simulink model "ADCS_Outline"  (R2019a)
settings: Solver=VariableStepAuto  StartTime=0.0  StopTime=duration  MaxStep=step
InitFcn:
  | SC_ODIN_INITIALIZATION
values from neighbouring files (symbols this model uses):
  A = [ v(1) v(4) v(5) v(7);        v(4) v(2) v(6) v(8);        v(5) v(6) v(3) v(9);        v(7) v(8) v(9) v(10) ]    [MagnetometerCalibration.m]    (also in SC_ODIN_INITIALIZATION.m = 0.06; test.m = asin(sin(N)/sin(n)*sin(a)))
  Amag = [0.910186583854  -0.00959593267728  0.00343590491018; -0.00959593267728  1.05471221352  0.0559849466324; 0.00343590491018  0.0559849466324  1.05528532305]    [MagnetometerBias.mat]    (also in MagnetometerCalibration.m = evecs/scale*evecs')
  argentina = [1612.36;-4182.16;-4522.83]    [SC_ODIN_INITIALIZATION.m]
  As = 0.2*0.3    (= 0.06)    [SC_ODIN_INITIALIZATION.m]
  b_mag = block.InputPort(3).Data    [MagnetometerCalibration.m]    (also in SC_ODIN_INITIALIZATION.m = [10;-15.5;-12.2]*1e-6)
  bmag = [1.00003671399e-05 -1.55007781395e-05 -1.22009762149e-05]    [MagnetometerBias.mat]    (also in MagnetometerCalibration.m = centerE)
  breakpoints = data(:,1)    [SC_ODIN_INITIALIZATION.m]
  c = 2.99792458e8    (= 299792458)    [SC_ODIN_INITIALIZATION.m]
  C_I = [0.045 0.0009 -0.00007;        0.0009 0.045 -0.00003;        -0.00007 -0.00003 0.009]    [SC_ODIN_INITIALIZATION.m]
  Cd = 2.0    (= 2)    [SC_ODIN_INITIALIZATION.m]
  controller_sample_rate = 0.5    [SC_ODIN_INITIALIZATION.m]
  D = [ 2 * x,            2 * y,            2 * z,            1 + 0 * x ]    [MagnetometerCalibration.m]    (also in SC_ODIN_INITIALIZATION.m = 0.01*[1;1;1])
  datapx = data(:,2)    [SC_ODIN_INITIALIZATION.m]
  datapy = data(:,3)    [SC_ODIN_INITIALIZATION.m]
  datapz = data(:,4)    [SC_ODIN_INITIALIZATION.m]
  datavx = data(:,5)    [SC_ODIN_INITIALIZATION.m]
  datavy = data(:,6)    [SC_ODIN_INITIALIZATION.m]
  datavz = data(:,7)    [SC_ODIN_INITIALIZATION.m]
  DCM_BT0 = eye(3)    [SC_ODIN_INITIALIZATION.m]
  G = 6.67408e-11    [SC_ODIN_INITIALIZATION.m]
  ground = [1266.06;-4295.81;4526.14]    [SC_ODIN_INITIALIZATION.m]
  I = [Ixx -Ixy -Ixz;      -Ixy Iyy -Iyz;      -Ixz -Iyz Izz]    [SC_ODIN_INITIALIZATION.m]
  invA_mag = block.InputPort(2).Data    [MagnetometerCalibration.m]    (also in SC_ODIN_INITIALIZATION.m = inv(Ellrot/scale*Ellrot'))
  JD_0 = start_day+start_fraction    [SC_ODIN_INITIALIZATION.m]
  Ks = 1367    [SC_ODIN_INITIALIZATION.m]
  L = [0.0000812 -0.0022136 -0.0225868]    [SC_ODIN_INITIALIZATION.m]
  Ls = 0.01*[-3; 3; 5]    [SC_ODIN_INITIALIZATION.m]
  M = 5.9722e24    (= 5.9722e+24)    [SC_ODIN_INITIALIZATION.m]    (also in visualisation.m = uicontrol('Style','text','String',{''},'Position',[710 100+2)
  magnetorquer_tau = 0.02    [SC_ODIN_INITIALIZATION.m]
  magnetorquer_x_saturation = 0.24    [SC_ODIN_INITIALIZATION.m]
  magnetorquer_y_saturation = 0.24    [SC_ODIN_INITIALIZATION.m]
  magnetorquer_z_saturation = 0.13    [SC_ODIN_INITIALIZATION.m]
  namibia = [5659.26;1238.85;-2659.2]    [SC_ODIN_INITIALIZATION.m]
  q = 0.6    [SC_ODIN_INITIALIZATION.m]
  radii = radii .* sgns    [MagnetometerCalibration.m]    (also in SC_ODIN_INITIALIZATION.m = [1;0.9;1.1])
  W0 = [1;0;1-1/240].*pi()/180    [SC_ODIN_INITIALIZATION.m]
  wheel_saturation = 0.23e-3    (= 0.00023)    [SC_ODIN_INITIALIZATION.m]
  wheel_tau = 2    [SC_ODIN_INITIALIZATION.m]
undefined symbols (not defined in the file or in its folder): DiscIntNeverNeededParam, nut80, sun_sensors
libraries: dspmathops x94, vrlib x70, dspsrcs4 x21, realtime_pacer_lib x1, dspsolvers x1, dspinverses x1
(part 4 of 6)

== matlab function ADCS_Outline/SGP4/SGP4 ==
  data: TT input; pos output size=3; vel output size=3
function [pos , vel] = SGP4(TT)
ge = 398600.8; % Earth gravitational constant
TWOPI = 2*pi;
MINUTES_PER_DAY = 1440.0;
MINUTES_PER_DAY_SQUARED = (MINUTES_PER_DAY * MINUTES_PER_DAY);
MINUTES_PER_DAY_CUBED = (MINUTES_PER_DAY * MINUTES_PER_DAY_SQUARED);

% TLE file
% ISS (ZARYA)             
% 1 25544U 98067A   19233.64704772  .00000489  00000-0  16413-4 0  9995
% 2 25544  51.6448  36.5251 0007392 309.8359 134.3211 15.50389354185417
tle1 = '1 25544U 98067A   19233.64704772  .00000489  00000-0  16413-4 0  9995';
tle2 = '2 25544  51.6448  36.5251 0007392 309.8359 134.3211 15.50389354185417';


% Open the TLE file and read TLE elements


% 19-32	04236.56031392	Element Set Epoch (UTC)
% 3-7	25544	Satellite Catalog Number
% 9-16	51.6335	Orbit Inclination (degrees)
% 18-25	344.7760	Right Ascension of Ascending Node (degrees)
% 27-33	0007976	Eccentricity (decimal point assumed)
% 35-42	126.2523	Argument of Perigee (degrees)
% 44-51	325.9359	Mean Anomaly (degrees)
% 53-63	15.70406856	Mean Motion (revolutions/day)
% 64-68	32890	Revolution Number at Epoch

    % read first line
    tline = tle1;

    Cnum = tline(3:7);      			        % Catalog Number (NORAD)
    SC   = tline(8);					        % Security Classification
    ID   = tline(10:17);			            % Identification Number
    epoch = str2double(tline(19:32));              % Epoch
    TD1   = str2double(tline(34:43));              % first time derivative
    TD2   = str2double(tline(45:50));              % 2nd Time Derivative
    ExTD2 = tline(51:52);                       % Exponent of 2nd Time Derivative
    BStar = str2double(tline(54:59));              % Bstar/drag Term
    ExBStar = str2double(tline(60:61));            % Exponent of Bstar/drag Term
    BStar = BStar*1e-5*10^ExBStar;
    Etype = tline(63);                          % Ephemeris Type
    Enum  = str2double(tline(65:end));             % Element Number
    
    % read second line
    tline = tle2;

    i = str2double(tline(9:16));                   % Orbit Inclination (degrees)
    raan = str2double(tline(18:25));               % Right Ascension of Ascending Node (degrees)
    e = 0.0007392 %str2double(strcat('0.',tline(27:33)));     % Eccentricity
    omega = str2double(tline(35:42));              % Argument of Perigee (degrees)
    M = str2double(tline(44:51));                  % Mean Anomaly (degrees)
    no = str2double(tline(53:63));                 % Mean Motion
    a = ( ge/(no*2*pi/86400)^2 )^(1/3);         % semi major axis (m)
    rNo = str2double(tline(64:68));                % Revolution Number at Epoch

satdata.epoch = epoch;
satdata.norad_number = Cnum;
satdata.bulletin_number = ID;
satdata.classification = SC; % almost always 'U'
satdata.revolution_number = rNo;
satdata.ephemeris_type = Etype;
satdata.xmo = M * (pi/180);
satdata.xnodeo = raan * (pi/180);
satdata.omegao = omega * (pi/180);
satdata.xincl = i * (pi/180);
satdata.eo = e;
satdata.xno = no * TWOPI / MINUTES_PER_DAY;
satdata.xndt2o = TD1 * 1e-8 * TWOPI / MINUTES_PER_DAY_SQUARED;
satdata.xndd6o = TD2 * TWOPI / MINUTES_PER_DAY_CUBED;
satdata.bstar = BStar;

tsince = (TT-58484-233.64704772)*MINUTES_PER_DAY; %epoch january 1st 2019 = 58484 MJD

[pos, vel] = sgp4(tsince, satdata);

function [pos, vel] = sgp4(tsince, satdata)

ae = 1.0;
tothrd = (2.0/3.0);
XJ3 = -2.53881e-6;
e6a = 1.0E-6;
xkmper = 6378.135;
ge = 398600.8; % Earth gravitational constant
CK2 = (1.0826158e-3 / 2.0);
CK4 = (-3.0 * -1.65597e-6 / 8.0);

% Constants
s = ae + 78 / xkmper;
qo = ae + 120 / xkmper;
xke = sqrt((3600.0 * ge) / (xkmper^3));
qoms2t = ((qo - s)^2)^2;
temp2 = xke / (satdata.xno);
a1 = temp2^tothrd;
cosio = cos (satdata.xincl);
theta2 = (cosio^2);
x3thm1 = 3.0 * theta2 - 1.0;
eosq = (satdata.eo^2);
betao2 = 1.0 - eosq;
betao = sqrt(betao2);
del1 = 1.5 * CK2 * x3thm1 / ((a1^2) * betao * betao2);
ao = a1 * ( 1.0 - del1*((1.0/3.0) + del1 * (1.0 + (134.0/81.0) * del1)));
delo = 1.5 * CK2 * x3thm1 / ((ao^2) * betao * betao2);
xnodp = (satdata.xno)/(1.0 + delo);
aodp = ao/(1.0 - delo);
% Initialization
% For perigee less than 220 kilometers, the isimp flag is set and
% the equations are truncated to linear variation in sqrt a and
% quadratic variation in mean anomaly.  Also, the c3 term, the
% delta omega term, and the delta m term are dropped.
isimp = 0;
if ((aodp * (1.0 - satdata.eo)/ ae) < (220.0/xkmper + ae))
    isimp = 1;
end
% For perigee below 156 km, the values of s and qoms2t are altered.
s4 = s;
qoms24 = qoms2t;
perige = (aodp * (1.0 - satdata.eo) - ae) * xkmper;
if (perige < 156)
    s4 = perige - 78.0;
    if (perige <= 98)
        s4 = 20.0;
    end
    qoms24 = (((120.0 - s4) * ae / xkmper)^4.0);
    s4 = s4 / xkmper + ae;
end
pinvsq = 1.0 / ( (aodp^2) * (betao2^2) );
tsi = 1.0 / (aodp - s4);
eta = aodp * (satdata.eo) * tsi;
etasq = (eta^2);
eeta = (satdata.eo) * eta;
psisq = abs( 1.0 - etasq);
coef = qoms24 * (tsi^4.0);
coef1 = coef / (psisq^3.5);
c2 = coef1 * xnodp * (aodp * (1.0 + 1.5 * etasq + eeta * (4.0 + etasq)) + 0.75 * CK2 * tsi / psisq * x3thm1 * (8.0 + 3.0 * etasq * (8.0 + etasq)));
c1 = (satdata.bstar) * c2;
sinio = sin(satdata.xincl);
a3ovk2 = -XJ3 / CK2 * (ae^3.0);
c3 = coef * tsi * a3ovk2 * xnodp * ae * sinio / (satdata.eo);
x1mth2 = 1.0 - theta2;
c4 = 2.0 * xnodp * coef1 * aodp * betao2 * ( eta * (2.0 + 0.5 * etasq) + (satdata.eo) * (0.5 + 2.0 * etasq) - 2.0 * CK2 * tsi / (aodp * psisq) * ( -3.0 * x3thm1 * ( 1.0 - 2.0 * eeta + etasq * (1.5 - 0.5*eeta)) + 0.75 * x1mth2 * (2.0 * etasq - eeta * (1.0 + etasq)) * cos(2.0 * (satdata.omegao))));
c5 = 2.0 * coef1 * aodp * betao2 * (1.0 + 2.75 * (etasq + eeta) + eeta * etasq);
theta4 = (theta2^2);
temp1 = 3.0 * CK2 * pinvsq * xnodp;
temp2 = temp1 * CK2 * pinvsq;
temp3 = 1.25 * CK4 * pinvsq * pinvsq * xnodp;
xmdot = xnodp + 0.5 * temp1 * betao * x3thm1 + 0.0625 * temp2 * betao * (13.0 - 78.0 * theta2 + 137.0 * theta4);
x1m5th = 1.0 - 5.0 * theta2;
omgdot = -0.5 * temp1 * x1m5th + 0.0625 * temp2 * (7.0 - 114.0 * theta2 + 395.0 * theta4) + temp3 * (3.0 - 36.0 * theta2 + 49.0 * theta4);
xhdot1 = -temp1 * cosio;
xnodot = xhdot1 + (0.5 * temp2 * (4.0 - 19.0 * theta2) + 2.0 * temp3 * (3.0 - 7.0 * theta2)) * cosio;
omgcof = (satdata.bstar) * c3 * cos(satdata.omegao);
xmcof = -(2.0/3.0) * coef * (satdata.bstar) * ae / eeta;
xnodcf = 3.5 * betao2 * xhdot1 * c1;
t2cof = 1.5 * c1;
xlcof = 0.125 * a3ovk2 * sinio * (3.0 + 5.0 * cosio) / (1.0 + cosio);
aycof = 0.25 * a3ovk2 * sinio;
delmo = ((1.0 + eta * cos(satdata.xmo))^3);
sinmo = sin(satdata.xmo);
x7thm1 = 7.0 * theta2 - 1.0;
if (isimp==0)	
    c1sq = (c1^2);
    d2 = 4.0 * aodp * tsi * c1sq;
    temp = d2 * tsi * c1 / 3.0;
    d3 = (17.0 * aodp + s4)*temp;
    d4 = 0.5 * temp * aodp * tsi * (221.0 * aodp + 31.0 * s4) * c1;
    t3cof = d2 + 2.0*c1sq;
    t4cof = 0.25 * (3.0 * d3 + c1 * (12.0 * d2 + 10.0 * c1sq));
    t5cof = 0.2 * (3.0 * d4 + 12.0 * c1 * d3 + 6.0 * d2 * d2 + 15.0 * c1sq * (2.0 * d2 + c1sq));
end
% Update for secular gravity and atmospheric drag.
xmdf = satdata.xmo + xmdot * tsince;
omgadf = satdata.omegao + omgdot * tsince;
xnoddf = satdata.xnodeo + xnodot * tsince;
omega = omgadf;
xmp = xmdf;
tsq = (tsince^2);
xnode = xnoddf + xnodcf * tsq;
tempa = 1.0 - c1 * tsince;
tempe = (satdata.bstar) * c4 * tsince;
templ = t2cof * tsq;
if (isimp == 0)
    delomg = omgcof * tsince;
    delm = xmcof*(((1.0 + eta * cos(xmdf))^ 3.0) - delmo);
    temp = delomg + delm;
    xmp = xmdf + temp;
    omega = omgadf - temp;
    tcube = tsq * tsince;
    tfour = tsince * tcube;
    tempa = tempa - d2 * tsq - d3 * tcube - d4 * tfour;
    tempe = tempe + (satdata.bstar) * c5 * (sin(xmp) - sinmo);
    templ = templ + t3cof * tcube + tfour * (t4cof + tsince * t5cof);
end
a = aodp * (tempa^2);
eo = (satdata.eo) - tempe;
xl = xmp + omega + xnode + xnodp*templ;
beta = sqrt(1.0 - (eo^2));
xn = xke / (a^1.5);
% Long period periodics
axn = eo * cos(omega);
temp = 1.0 / (a * (beta^2));
xll = temp * xlcof * axn;
aynl = temp * aycof;
xlt = xl + xll;
ayn = eo * sin(omega) + aynl;
% Solve Kepler's Equation
capu = modulus(xlt - xnode,2*pi);
temp2 = capu;
count=1;
while(1)
    sinepw = sin(temp2);
    cosepw = cos(temp2);
    temp3 = axn * sinepw;
    temp4 = ayn * cosepw;
    temp5 = axn * cosepw;
    temp6 = ayn * sinepw;
    epw = (capu - temp4 + temp3 - temp2) / (1.0 - temp5 - temp6) + temp2;
    temp7 = temp2;
    temp2 = epw;
    count = count+1;
	if ((count>10) || (abs(epw - temp7) <= e6a))
		break
	end
end

% Short period preliminary quantities
ecose = temp5 + temp6;
esine = temp3 - temp4;
elsq = (axn^2) + (ayn^2);
temp = 1.0 - elsq;
pl = a * temp;
r = a * (1.0 - ecose);
temp1 = 1.0 / r;
rdot = xke * sqrt(a) * esine * temp1;
rfdot = xke * sqrt(pl) * temp1;
temp2 = a * temp1;
betal = sqrt(temp);
temp3 = 1.0 / (1.0 + betal);
cosu = temp2 * (cosepw - axn + ayn * esine * temp3);
sinu = temp2 * (sinepw - ayn - axn * esine * temp3);
u = actan(sinu, cosu);
sin2u = 2.0 * sinu * cosu;
cos2u = 2.0 * (cosu^2) - 1.0;
temp = 1.0 / pl;
temp1 = CK2 * temp;
temp2 = temp1 * temp;
% Update for short periodics
rk = r * (1.0 - 1.5 * temp2 * betal * x3thm1) + 0.5 * temp1 * x1mth2 * cos2u;
uk = u - 0.25 * temp2 * x7thm1 * sin2u;
xnodek = xnode + 1.5 * temp2 * cosio * sin2u;
xinck = (satdata.xincl) + 1.5 * temp2 * cosio * sinio * cos2u;
rdotk = rdot - xn * temp1 * x1mth2 * sin2u;
rfdotk = rfdot + xn * temp1 * (x1mth2 * cos2u + 1.5 * x3thm1);
% Orientation vectors
MV.v(1) = -sin(xnodek) * cos(xinck);
MV.v(2) = cos(xnodek) * cos(xinck);
MV.v(3) = sin(xinck);

NV.v(1) = cos(xnodek);
NV.v(2) = sin(xnodek);
NV.v(3) = 0;

for count=1:3
	UV.v(count) = MV.v(count) * sin(uk) + NV.v(count) * cos(uk);
	VV.v(count) = MV.v(count) * cos(uk) - NV.v(count) * sin(uk);
end

% position + velocity
for count=1:3
	pos.v(count) = rk * UV.v(count);
	vel.v(count) = rdotk * UV.v(count) + rfdotk * VV.v(count);
end
xkmper = 6378.135;

for count=1:3
    pos(count) = pos.v(count) * xkmper;
    vel(count) = vel.v(count) * xkmper / 60;
end



function modu = modulus(arg1, arg2)

modu = arg1 - floor(arg1/arg2) * arg2;

if (modu >= 0)
    return
else
    modu = modu + arg2;
    return
end
function t = actan(y, x)

t = atan2(y,x);
if (t < 0)
    t = t + 2*pi;
end

== matlab function ADCS_Outline/TEME to ITRF/From David Vallado ==
  data: steme input; secef output; rteme input; recef output; vteme input; ateme input; ttt input; jdut1 input; lod input; xp input; yp input; eqeterms input; vecef output; aecef output; DCM_ET output
% ----------------------------------------------------------------------------
%
%                           function teme2ecef
%
%  this function trsnforms a vector from the true equator mean equniox frame
%    (teme), to an earth fixed (ITRF) frame.  the results take into account
%    the effects of sidereal time, and polar motion.
%
%  author        : david vallado                  719-573-2600   30 oct 2017
%
%  revisions
%
%  inputs          description                    range / units
%    rteme       - position vector teme           km
%    steme       - another position vector teme   km
%    vteme       - velocity vector teme           km/s
%    ateme       - acceleration vector teme       km/s2
%    ttt         - julian centuries of tt         centuries
%    jdut1       - julian date of ut1             days from 4713 bc
%    lod         - excess length of day           sec
%    xp          - polar motion coefficient       rad
%    yp          - polar motion coefficient       rad
%    eqeterms    - use extra two terms (kinematic) after 1997  0, 2
%
%  outputs       :
%    recef       - position vector earth fixed    km
%    secef       - another position vector earth fixed    km
%    vecef       - velocity vector earth fixed    km/s
%    aecef       - acceleration vector earth fixedkm/s2
%
%  locals        :
%    st          - matrix for pef - tod 
%    pm          - matrix for ecef - pef 
%
%  coupling      :
%   gstime       - greenwich mean sidereal time   rad
%   polarm       - rotation for polar motion      pef - ecef
%
%  references    :
%    vallado       2013, 231-233
%
% [recef, vecef, aecef] = teme2ecef( rteme, vteme, ateme, ttt, jdut1, lod, xp, yp, eqeterms );
% ----------------------------------------------------------------------------

function [secef, recef, vecef, aecef, DCM_ET] = teme2ecef(steme, rteme, vteme, ateme, ttt, jdut1, lod, xp, yp, eqeterms )

        deg2rad = pi/180.0;
        
        
        % ------------------------ find gmst --------------------------
        gmst= gstime( jdut1 );

        % find omega from nutation theory
        omega=  125.04452222  + (   -6962890.5390 *ttt + ...
                7.455 *ttt*ttt + 0.008 *ttt*ttt*ttt )  / 3600.0;
        omega= rem( omega, 360.0  ) * deg2rad;
        
        % ------------------------ find mean ast ----------------------
        % teme does not include the geometric terms here
        % after 1997, kinematic terms apply
        if (jdut1 > 2450449.5 ) && (eqeterms > 0)
            gmstg = gmst ...
                   + 0.00264*pi /(3600*180)*sin(omega) ...
                   + 0.000063*pi /(3600*180)*sin(2.0 *omega);
        else
            gmstg = gmst;
        end

        gmstg = rem (gmstg, 2.0*pi);

        st = zeros(3,3);
        st(1,1) =  cos(gmstg);
        st(1,2) = -sin(gmstg);
        st(1,3) =  0.0;
        st(2,1) =  sin(gmstg);
        st(2,2) =  cos(gmstg);
        st(2,3) =  0.0;
        st(3,1) =  0.0;
        st(3,2) =  0.0;
        st(3,3) =  1.0;

        [pm] = polarm(xp,yp,ttt,'80');

        rpef  = st'*rteme;
        recef = pm'*rpef;
 
        spef  = st'*steme;
        secef = pm'*spef;

        thetasa    = 7.29211514670698e-05 * (1.0  - lod/86400.0 );
        omegaearth = [0; 0; thetasa;];

        vpef  = st'*vteme - cross( omegaearth,rpef );
        vecef = pm'*vpef;

        temp  = cross(omegaearth,rpef);

        aecef = pm'*(st'*ateme - cross(omegaearth,temp) ...
                - 2.0*cross(omegaearth,vpef));
        DCM_ET = pm'*st;

%fprintf(1,'st gmst %11.8f ast %11.8f ome  %11.8f \n', gmst*180/pi, ast*180/pi, omegaearth*180/pi );
% -----------------------------------------------------------------------------
%
%                           function gstime
%
%  this function finds the greenwich sidereal time (iau-82).
%
%  author        : david vallado                  719-573-2600    7 jun 2002
%
%  revisions
%                -
%
%  inputs          description                    range / units
%    jdut1       - julian date of ut1             days from 4713 bc
%
%  outputs       :
%    gst         - greenwich sidereal time        0 to 2pi rad
%
%  locals        :
%    temp        - temporary variable for reals   rad
%    tut1        - julian centuries from the
%                  jan 1, 2000 12 h epoch (ut1)
%
%  coupling      :
%
%  references    :
%    vallado       2007, 193, Eq 3-43
%
% gst = gstime(jdut1);
% -----------------------------------------------------------------------------

function gst = gstime(jdut1)

        twopi      = 2.0*pi;
        deg2rad    = pi/180.0;

        % ------------------------  implementation   ------------------
        tut1= ( jdut1 - 2451545.0 ) / 36525.0;

        temp = - 6.2e-6 * tut1 * tut1 * tut1 + 0.093104 * tut1 * tut1  ...
               + (876600.0 * 3600.0 + 8640184.812866) * tut1 + 67310.54841;

        % 360/86400 = 1/240, to deg, to rad
        temp = rem( temp*deg2rad/240.0,twopi );

        % ------------------------ check quadrants --------------------
        if ( temp < 0.0 )
            temp = temp + twopi;
        end

        gst = temp;

%�
% ----------------------------------------------------------------------------
%
%                           function polarm
%
%  this function calulates the transformation matrix that accounts for polar
%    motion. both the 1980 and 2000 theories are handled. note that the rotation 
%    order is different between 1980 and 2000 .
%
%  author        : david vallado                  719-573-2600   25 jun 2002
%
%  revisions
%    vallado     - consolidate with iau 2000                     14 feb 2005
%
%  inputs          description                    range / units
%    xp          - polar motion coefficient       rad
%    yp          - polar motion coefficient       rad
%    ttt         - julian centuries of tt (00 theory only)
%    opt         - method option                  '01', '02', '80'
%
%  outputs       :
%    pm          - transformation matrix for ecef - pef
%
%  locals        :
%    convrt      - conversion from arcsec to rad
%    sp          - s prime value
%
%  coupling      :
%    none.
%
%  references    :
%    vallado       2004, 207-209, 211, 223-224
%
% [pm] = polarm ( xp, yp, ttt, opt );
% ----------------------------------------------------------------------------

function [pm] = polarm ( xp, yp, ttt, opt )


        cosxp = cos(xp);
        sinxp = sin(xp);
        cosyp = cos(yp);
        sinyp = sin(yp);

        if (opt == '80')
            pm = zeros(3,3);
            pm(1,1) =  cosxp;
            pm(1,2) =  0.0;
            pm(1,3) = -sinxp;
            pm(2,1) =  sinxp * sinyp;
            pm(2,2) =  cosyp;
            pm(2,3) =  cosxp * sinyp;
            pm(3,1) =  sinxp * cosyp;
            pm(3,2) = -sinyp;
            pm(3,3) =  cosxp * cosyp;

            % a1 = rot2mat(xp);
            % a2 = rot1mat(yp);
            % pm = a2*a1;          
            % Approximate matrix using small angle approximations
            %pm(1,1) =  1.0;
            %pm(2,1) =  0.0;
            %pm(3,1) =  xp;
            %pm(1,2) =  0.0;
            %pm(2,2) =  1.0;
            %pm(3,2) = -yp;
            %pm(1,3) = -xp;
            %pm(2,3) =  yp;
            %pm(3,3) =  1.0;
        else  
            convrt = pi / (3600.0*180.0);
            % approximate sp value in rad
            sp = -47.0e-6 * ttt * convrt;
            cossp = cos(sp);
            sinsp = sin(sp);

            % form the matrix
            pm = zeros(3,3);
            pm(1,1) =  cosxp * cossp;
            pm(1,2) = -cosyp * sinsp + sinyp * sinxp * cossp;
            pm(1,3) = -sinyp * sinsp - cosyp * sinxp * cossp;
            pm(2,1) =  cosxp * sinsp;
            pm(2,2) =  cosyp * cossp + sinyp * sinxp * sinsp;
            pm(2,3) =  sinyp * cossp - cosyp * sinxp * sinsp;
            pm(3,1) =  sinxp;
            pm(3,2) = -sinyp * cosxp;
            pm(3,3) =  cosyp * cosxp;

            % a1 = rot1mat(yp);
            % a2 = rot2mat(xp);
            % a3 = rot3mat(-sp);
            % pm = a3*a2*a1;
        end

== matlab function ADCS_Outline/IGRF/MATLAB Function1 ==
  data: X input; lat output; Y input; Z input; lon output; altitude output; h output
function [lat,lon,altitude,h]=xyz2ell3(X,Y,Z)
% XYZ2ELL3  Converts cartesian coordinates to ellipsoidal.
%   Uses direct algorithm in B.R. Bowring, "The accuracy of
%   geodetic latitude and height equations", Survey
%   Review, v28 #218, October 1985, pp.202-206.  Vectorized.
%   See also XYZ2ELL, XYZ2ELL2.
% Version: 2011-02-19
% Usage:   [lat,lon,h]=xyz2ell3(X,Y,Z,a,b,e2)
%          [lat,lon,h]=xyz2ell3(X,Y,Z)
% Input:   X \
%          Y  > vectors of cartesian coordinates in CT system (m)
%          Z /
%          a   - ref. ellipsoid major semi-axis (m); default GRS80
%          b   - ref. ellipsoid minor semi-axis (m); default GRS80
%          e2  - ref. ellipsoid eccentricity squared; default GRS80
% Output:  lat - vector of ellipsoidal latitudes (radians)
%          lon - vector of ellipsoidal longitudes (radians)
%          h   - vector of ellipsoidal heights (m)

% Copyright (c) 2011, Michael R. Craymer
% All rights reserved.
% Email: mike@craymer.com
% 
% if nargin ~= 3 & nargin ~= 6
%   warning('Incorrect number of input arguments');
%   return
% end
% if nargin == 3
  [a,b,e2]=refell('grs80');
% end

lon=atan2(Y,X);
e=e2*(a/b)^2;
p=sqrt(X.*X+Y.*Y);
r=sqrt(p.*p+Z.*Z);
u=atan(b.*Z.*(1+e.*b./r)./(a.*p));
lat=atan((Z+e.*b.*sin(u).^3)./(p-e2.*a.*cos(u).^3));
v=a./sqrt(1-e2.*sin(lat).^2);
h=p.*cos(lat)+Z.*sin(lat)-a*a./v;
altitude = r;



%complement function
function [a,b,e2,finv]=refell(type)
% REFELL  Computes reference ellispoid parameters.
%   Reference: Department of Defence World Geodetic
%   System 1984, DMA TR 8350.2, 1987.
%   TOPEX Reference: <http://topex-www.jpl.nasa.gov/aviso/text/general/news/hdbk311.htm#CH3.3>
% Version: 1 Jun 04
% Usage:   [a,b,e2,finv]=refell(type)
% Input:   type - reference ellipsoid type (char)
%                 CLK66 = Clarke 1866
%                 GRS67 = Geodetic Reference System 1967
%                 GRS80 = Geodetic Reference System 1980
%                 WGS72 = World Geodetic System 1972
%                 WGS84 = World Geodetic System 1984
%                 ATS77 = Quasi-earth centred ellipsoid for ATS77
%                 NAD27 = North American Datum 1927 (=CLK66)
%                 NAD83 = North American Datum 1927 (=GRS80)
%                 INTER = International
%                 KRASS = Krassovsky (USSR)
%                 MAIRY = Modified Airy (Ireland 1965/1975)
%                 TOPEX = TOPEX/POSEIDON ellipsoid
% Output:  a    - major semi-axis (m)
%          b    - minor semi-axis (m)
%          e2   - eccentricity squared
%          finv - inverse of flattening

% Copyright (c) 2011, Michael R. Craymer
% All rights reserved.
% Email: mike@craymer.com

type=upper(type);
if (type=='CLK66' | type=='NAD27')
  a=6378206.4;
  finv=294.9786982;
elseif type=='GRS67'
  a=6378160.0;
  finv=298.247167427;
elseif (type=='GRS80' | type=='NAD83')
  a=6378137.0;
  finv=298.257222101;
elseif (type=='WGS72')
  a=6378135.0;
  finv=298.26;
elseif (type=='WGS84')
  a=6378137.0;
  finv=298.257223563;
elseif type=='ATS77'
  a=6378135.0;
  finv=298.257;
elseif type=='KRASS'
  a=6378245.0;
  finv=298.3;
elseif type=='INTER'
  a=6378388.0;
  finv=297.0;
elseif type=='MAIRY'
  a=6377340.189;
  finv=299.3249646;
elseif type=='TOPEX'
  a=6378136.3;
  finv=298.257;
end
f=1/finv;
b=a*(1-f);
e2=1-(1-f)^2;

== matlab function ADCS_Outline/IGRF/MATLAB Function2 ==
  data: dx input; dX output; dy input; dz input; lat input; lon input; dY output; dZ output
function [dX,dY,dZ]=lg2ct(dx,dy,dz,lat,lon)
% LG2CT  Converts local geodetic coordinate differences to CT.
%   Local origin at lat,lon,h. If lat,lon are vectors, dx,dy,dz
%   are referenced to orgin at lat,lon of same index. If
%   astronomic lat,lon input, output is in local astronomic
%   system. Vectorized in both dx,dy,dz and lat,lon. See also
%   CT2LG.
% Version: 2013-02-12
% Usage:   [dX,dY,dZ]=lg2ct(dx,dy,dz,lat,lon)
% Input:   dx  - vector of x coordinates in local system (north)
%          dy  - vector of y coordinates in local system (east)
%          dz  - vector of z coordinates in local system (ht)
%          lat - lat(s) of local system origin (rad); may be vector
%          lon - lon(s) of local system origin (rad); may be vector
% Output:  dX  - vector of X coordinate differences in CT
%          dY  - vector of Y coordinate differences in CT
%          dZ  - vector of Z coordinate differences in CT

% Copyright (c) 2013, Michael R. Craymer
% All rights reserved.
% Email: mike@craymer.com

if nargin ~= 5
  warning('Incorrect number of input arguments');
  return
end

n=length(dx);
if length(lat)==1
  lat=ones(n,1)*lat;
  lon=ones(n,1)*lon;
end
R=zeros(3,3,n);

R(1,1,:)=-sin(lat').*cos(lon');
R(2,1,:)=-sin(lat').*sin(lon');
R(3,1,:)=cos(lat');
R(1,2,:)=-sin(lon');
R(2,2,:)=cos(lon');
R(3,2,:)=zeros(1,n);
R(1,3,:)=cos(lat').*cos(lon');
R(2,3,:)=cos(lat').*sin(lon');
R(3,3,:)=sin(lat');

RR=reshape(R(1,:,:),3,n);
dX=sum(RR'.*[dx dy dz],2);
RR=reshape(R(2,:,:),3,n);
dY=sum(RR'.*[dx dy dz],2);
RR=reshape(R(3,:,:),3,n);
dZ=sum(RR'.*[dx dy dz],2);

== matlab function ADCS_Outline/Sun/MATLAB Function1 ==
  data: rmod input; reci output; ttt input
%                           function mod2eci
%
%  this function transforms a vector from the mean equator mean equinox of
%    date (mod) to the mean equator mean equinox (j2000) frame.
%
%  author        : david vallado                  719-573-2600   25 jun 2002
%
%  revisions
%    vallado     - consolidate with iau 2000                     14 feb 2005
%
%  inputs          description                    range / units
%    rmod        - position vector of date
%                    mean equator, mean equinox   km
%    vmod        - velocity vector of date
%                    mean equator, mean equinox   km/s
%    amod        - acceleration vector of date
%                    mean equator, mean equinox   km/s2
%    ttt         - julian centuries of tt         centuries
%
%  outputs       :
%    reci        - position vector eci            km
%    veci        - velocity vector eci            km/s
%    aeci        - acceleration vector eci        km/s2
%
%  locals        :
%    none.
%
%  coupling      :
%   precess      - rotation for precession        mod - eci
%
%  references    :
%    vallado       2001, 219-220, eq 3-68
%
% [reci,veci,aeci] = mod2eci  ( rmod,vmod,amod,ttt );
% ----------------------------------------------------------------------------

function reci  = mod2eci  ( rmod,ttt )

        prec = zeros(3,3);
        [prec,psia,wa,ea,xa] = precess ( ttt );

        reci = prec*rmod;
%�
% ----------------------------------------------------------------------------
%
%                           function precess
%
%  this function calulates the transformation matrix that accounts for the effects
%    of precession. both the 1980 and 2000 theories are handled. note that the 
%    required parameters differ a little. 
%
%  author        : david vallado                  719-573-2600   25 jun 2002
%
%  revisions
%    vallado     - consolidate with iau 2000                     14 feb 2005
%
%  inputs          description                    range / units
%    ttt         - julian centuries of tt
%    opt         - method option                  '01', '02', '96', '80'
%
%  outputs       :
%    prec        - transformation matrix for mod - j2000 (80 only)
%    psia        - cannonical precession angle    rad    (00 only)
%    wa          - cannonical precession angle    rad    (00 only)
%    ea          - cannonical precession angle    rad    (00 only)
%    xa          - cannonical precession angle    rad    (00 only)
%
%  locals        :
%    ttt2        - ttt squared
%    ttt3        - ttt cubed
%    zeta        - precession angle               rad
%    z           - precession angle               rad
%    theta       - precession angle               rad
%    oblo        - obliquity value at j2000 epoch "%
%
%  coupling      :
%    none        -
%
%  references    :
%    vallado       2004, 214-216, 219-221
%
% [prec,psia,wa,ea,xa] = precess ( ttt, opt );
% ----------------------------------------------------------------------------

function [prec,psia,wa,ea,xa] = precess ( ttt );

       % sethelp;
        
        % " to rad
        convrt = pi / (180.0*3600.0);
        ttt2= ttt * ttt;
        ttt3= ttt2 * ttt;

        % ------------------- fk4 b1950 precession angles --------------------
%         if (opt == '50')
% 
%             % ---- Seidelmann pg 107             
%             % for these calls, ttt will come in with the current jd
% %            t1= 0.0; %(ttt - 2433282.42345905)/365242.198782;  % set start as B1850, 0.0 to simplify
% %            t2= (ttt - 2396758.203)/365242.198782;  % uses B1850
% %            ttt = t2 - t1;
% %            ttt2 = ttt * ttt;
% %            ttt3 = ttt * ttt2;
% %            fprintf(1,'50prec %15.9f  \n',ttt);
%             % exp supp 61 pg 38
% %            psia = 50.3708 + 0.0050 * ttt;
% %            wa = 0.0;
% %            ea = 0.0;
% %            xa = 0.1247 - 0.0188 * ttt;
% %            zeta =  (23035.545 + 139.720*t1 + 0.060 *t1*t1)*ttt + (30.240-0.270*t1)*ttt2 + 17.995*ttt3; % "
% %            theta=  (20051.12 - 85.29*t1 - 0.37 *t1*t1)*ttt + (-42.65-0.37*t1)*ttt2 - 41.80*ttt3;
% %            z    =  (23035.545 + 139.720*t1 + 0.060 *t1*t1)*ttt + (109.480+0.390*t1)*ttt2 + 18.325*ttt3;
% 
%             % ---- Newcomb Exp Supp 61 approach, but see GTDS pg 3-17
%             % Exp Supp 61 says use 1900? but gtds says use 1950. 
%             % for these calls, ttt will come in with the current jd
%             t1= 0.0; %(ttt - 2415020.31352)/36524.2198782;  % set start as B1900, 0.0 to simplify
% %            t2= (ttt - 2415020.31352)/36525;  % uses B1900   
%             t2= (ttt - 2433282.42345905)/36525;  % uses B1950  
% %            ttt = t2 - t1;
% %            ttt2 = ttt * ttt;
% %            ttt3 = ttt * ttt2;
%             % exp supp 61 pg 38
%             psia = 50.3708 + 0.0050 * ttt;
%             wa = 0.0; % not sure which one is which...
%             ea = 84428.26 -   46.845*ttt - 0.00059*ttt2 + 0.00181*ttt3;
%             xa = 0.1247 - 0.0188 * ttt;
%            fprintf(1,'50prec %15.9f  \n',ttt);
%            % seems like Exp supp 61 is ok with 1900 as epoch, and Seidlemann is ok with listed measr,  
% %            zeta =  (2304.25 + 1.396*t1)*ttt + 0.302*ttt2 + 0.018*ttt3; % "
% %            theta=  (2004.682 - 0.853*t1)*ttt -0.426*ttt2 - 0.042*ttt3;
% %            z    =  (2304.25 + 1.396*t1)*ttt + 1.093*ttt2 + 0.018*ttt3;
%             % GTDS pg 3-17 using days from 1950 - avoids long rpecession
%             % constants...
%             zeta =  2304.9969*ttt + 0.302*ttt2 + 0.01808*ttt3; % "
%             theta=  2004.2980*ttt -0.425936*ttt2 - 0.0416*ttt3;
%             z    =  2304.9969*ttt + 1.092999*ttt2 + 0.0192*ttt3;
%             
% 
%             % tp-008 36-45
%             % ttt is tropical centruies from 1950 36524.22 days
%             prec = zeros(3,3);
%             prec(1,1) =  1.0 - 2.9696e-4 * ttt2 - 1.3e-7 * ttt3;
%             prec(1,2) =  2.234941e-2 * ttt + 6.76e-6 * ttt2 - 2.21e-6 * ttt3;
%             prec(1,3) =  9.7169e-3 * ttt - 2.07e-6 * ttt2 - 9.6e-7 * ttt3;
%             prec(2,1) =  -prec(1,2);
%             prec(2,2) =  1.0 - 2.4975e-4 * ttt2 - 1.5e-7 * ttt3;
%             prec(2,3) =  - 1.0858e-4 * ttt2;
%             prec(3,1) =  -prec(1,3);
%             prec(3,2) =  prec(2,3);
%             prec(3,3) =  1.0 - 4.721e-5 * ttt2;
%  
%             
%            % pass these back out for testing
%            psia = zeta;
%            wa = theta;
%            ea = z;
%         % ------------------- iau 76 precession angles --------------------
%         else
%           if (opt == '80')
%     fprintf(1,'80prec %15.9f  \n',ttt);
            psia =             5038.7784*ttt - 1.07259*ttt2 - 0.001147*ttt3; % "
            wa   = 84381.448                 + 0.05127*ttt2 - 0.007726*ttt3;
            ea   = 84381.448 -   46.8150*ttt - 0.00059*ttt2 + 0.001813*ttt3;
            xa   =               10.5526*ttt - 2.38064*ttt2 - 0.001125*ttt3;
            zeta =             2306.2181*ttt + 0.30188*ttt2 + 0.017998*ttt3; % "
            theta=             2004.3109*ttt - 0.42665*ttt2 - 0.041833*ttt3;
            z    =             2306.2181*ttt + 1.09468*ttt2 + 0.018203*ttt3;
          % ------------------ iau 03 precession angles -------------------
%           else
%             oblo =  84381.406; % "
%             psia =  (((( -0.0000000951 * ttt + 0.000132851 ) * ttt - 0.00114045 ) * ttt - 1.0790069 ) * ttt + 5038.481507 ) * ttt; % "
%             wa   =  ((((  0.0000003337 * ttt - 0.000000467 ) * ttt - 0.00772503 ) * ttt + 0.0512623 ) * ttt -    0.025754 ) * ttt + oblo;
%             ea   =  (((( -0.0000000434 * ttt - 0.000000576 ) * ttt + 0.00200340 ) * ttt - 0.0001831 ) * ttt -   46.836769 ) * ttt + oblo;
%             xa   =  (((( - 0.0000000560 * ttt + 0.000170663 ) * ttt - 0.00121197 ) * ttt - 2.3814292 ) * ttt +   10.556403 ) * ttt;
% 
%             zeta =  (((( - 0.0000003173 * ttt - 0.000005971 ) * ttt + 0.01801828 ) * ttt + 0.2988499 ) * ttt + 2306.083227 ) * ttt + 2.650545; % "
%             theta=  (((( - 0.0000001274 * ttt - 0.000007089 ) * ttt - 0.04182264 ) * ttt - 0.4294934 ) * ttt + 2004.191903 ) * ttt;
%             z    =  ((((   0.0000002904 * ttt - 0.000028596 ) * ttt + 0.01826837 ) * ttt + 1.0927348 ) * ttt + 2306.077181 ) * ttt - 2.650545;
%           end;
%         end;
        
        % convert units to rad
        psia = psia  * convrt; % rad
        wa   = wa    * convrt;
        ea   = ea    * convrt;
        xa   = xa    * convrt;
        zeta = zeta  * convrt; 
        theta= theta * convrt;
        z    = z     * convrt;
%iauhelp='y';         
%fprintf(1,'pr %11.7f  %11.7f  %11.7fdeg \n',zeta*180/pi,theta*180/pi,z*180/pi );
%         if (iauhelp == 'y')
%             fprintf(1,'pr %11.7f  %11.7f  %11.7f %11.7fdeg \n',psia*180/pi,wa*180/pi,ea*180/pi,xa*180/pi );
%             fprintf(1,'pr %11.7f  %11.7f  %11.7fdeg \n',zeta*180/pi,theta*180/pi,z*180/pi );
%         end;
% 
%         if (strcmp(opt,'80')==1) % || (strcmp(opt,'50') == 1)
            coszeta  = cos(zeta);
            sinzeta  = sin(zeta);
            costheta = cos(theta);
            sintheta = sin(theta);
            cosz     = cos(z);
            sinz     = sin(z);

            % ----------------- form matrix  mod to j2000 -----------------
            prec = zeros(3,3);
            prec(1,1) =  coszeta * costheta * cosz - sinzeta * sinz;
            prec(1,2) =  coszeta * costheta * sinz + sinzeta * cosz;
            prec(1,3) =  coszeta * sintheta;
            prec(2,1) = -sinzeta * costheta * cosz - coszeta * sinz;
            prec(2,2) = -sinzeta * costheta * sinz + coszeta * cosz;
            prec(2,3) = -sinzeta * sintheta;
            prec(3,1) = -sintheta * cosz;
            prec(3,2) = -sintheta * sinz;
            prec(3,3) =  costheta;

            % ----------------- do rotations instead ----------------------
            % p1 = rot3mat( z );
            % p2 = rot2mat( -theta );
            % p3 = rot3mat( zeta );
            % prec = p3*p2*p1;
%         elseif (strcmp(opt,'50') ~= 1)
%             oblo = oblo * convrt; % " to rad
%             a4  = rot3mat(-xa);
%             a5  = rot1mat(wa);
%             a6  = rot3mat(psia);
%             a7  = rot1mat(-oblo);
%             prec = a7*a6*a5*a4;
%            % prec = zeros(3);
%         end;
